simulink model "hw1_first_order"  (R2014b)
settings: Solver=ode45  StartTime=0.0  StopTime=10.0  RelTol=1e-3
settings Model: Creator=kjartan  LastModifiedBy=kjartan

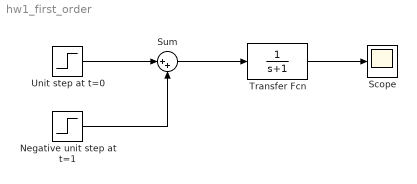
== system hw1_first_order ==
  Negative unit step at t=1 : Step  After=-1  SampleTime=0
  Scope : Scope
  Sum : Sum  Inputs=|++
  Transfer Fcn : TransferFcn  Denominator=[1 1]
  Unit step at t=0 : Step  Time=0  SampleTime=0
  wires:
  Sum/1 -> Transfer Fcn/1
  Unit step at t=0/1 -> Sum/1
  Negative unit step at t=1/1 -> Sum/2
  Transfer Fcn/1 -> Scope/1
